simulink model "exp8_2"  (R2023a)
settings: Solver=VariableStepAuto  StartTime=0.0  StopTime=8.0  RelTol=1e-3
settings Model: Creator=Lenovo  LastModifiedBy=zt

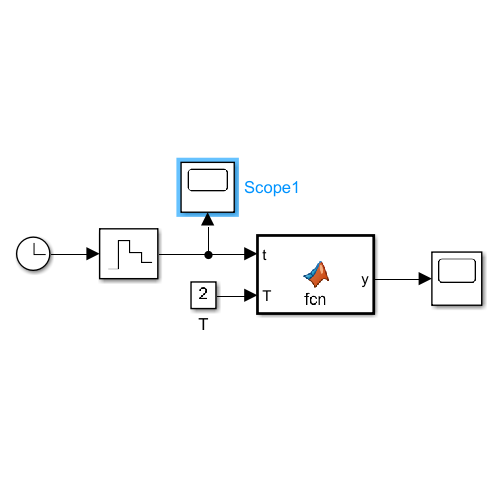
[thumbnail: Simulink's stored preview of the top-level diagram]
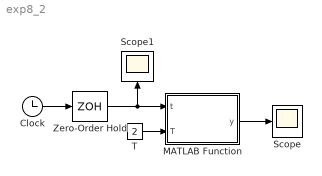
== system exp8_2 ==
  Clock : Clock
      settings: Decimation=8
  MATLAB Function : MATLAB Function  TreatAsAtomicUnit=on
  Scope : Scope
  Scope1 : Scope
  T : Constant  Value=2
  Zero-Order Hold : ZeroOrderHold  SampleTime=1/1000
  wires:
  T/1 -> MATLAB Function/2(T)
  Clock/1 -> Zero-Order Hold/1
  MATLAB Function/1(y) -> Scope/1
  Zero-Order Hold/1 -> MATLAB Function/1(t), Scope1/1

== matlab function exp8_2/MATLAB Function ==
  data: t input; y output; T input
function y = fcn(t, T)
    if t >= 0 && t < T
        y = t^2;
    elseif t >= T && t < 2*T
        y = (2*T - t)^2;
    else
        y = 0;
    end
end
